simulink model "Vehicle_direction_detection"  (R2019a)
settings: Solver=FixedStepAuto  StartTime=0.0  StopTime=2000  FixedStep=0.01  RelTol=1e-3
libraries: simulink x6
settings Model: DataDictionary=Vehicle_Direction_Detection.sldd  Creator=賽維涅什  LastModifiedBy=賽維涅什
settings OptimizationCC: DefaultParameterBehavior=Inlined  EnhancedBackFolding=on  PassReuseOutputArgsAs=Individual arguments  OptimizeBlockOrder=speed  DifferentSizesBufferReuse=on  OptimizationCustomize=off
settings DebuggingCC: ParameterTunabilityLossMsg=error
settings SFSimCC: MATLABDynamicMemAlloc=off
settings RTWCC: SystemTargetFile=ert.tlc  GenCodeOnly=on  TemplateMakefile=ert_default_tmf  GenerateReport=on  IncludeHyperlinkInReport=on  LaunchReport=on  GenerateTraceInfo=on  GenerateTraceReport=on  GenerateTraceReportSl=on  GenerateTraceReportSf=on  GenerateTraceReportEml=on
settings CodeAppCC: ForceParamTrailComments=on  IgnoreCustomStorageClasses=off  OperatorAnnotations=on  SimulinkDataObjDesc=on  SFDataObjDesc=on  InsertBlockDesc=on
settings ERTTargetCC: TargetLangStandard=C99 (ISO)  GenerateSampleERTMain=on  InlinedParameterPlacement=NonHierarchical  ERTCustomFileTemplate=example_file_process.tlc

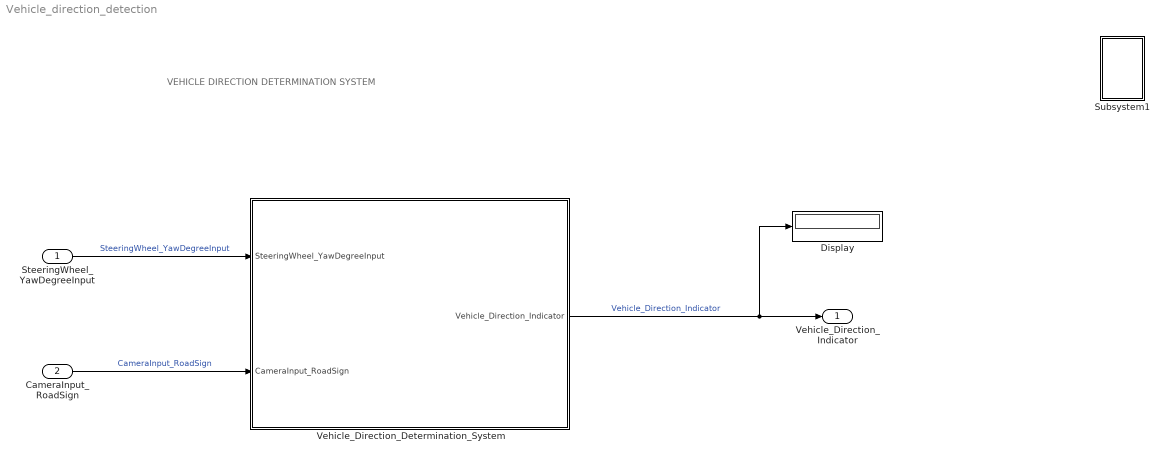
== system Vehicle_direction_detection ==
  note: VEHICLE DIRECTION DETERMINATION SYSTEM
  SteeringWheel_YawDegreeInput : Inport
  CameraInput_RoadSign : Inport  Port=2
  " Vehicle_Direction_Determination_System" : Subsystem
  Display : Display
  Subsystem1 : Subsystem
  Vehicle_Direction_Indicator : Outport
  wires:
  SteeringWheel_YawDegreeInput/1 -> " Vehicle_Direction_Determination_System"/1(SteeringWheel_YawDegreeInput)  "SteeringWheel_YawDegreeInput"
  CameraInput_RoadSign/1 -> " Vehicle_Direction_Determination_System"/2(CameraInput_RoadSign)  "CameraInput_RoadSign"
  " Vehicle_Direction_Determination_System"/1(Vehicle_Direction_Indicator) -> Display/1, Vehicle_Direction_Indicator/1  "Vehicle_Direction_Indicator"

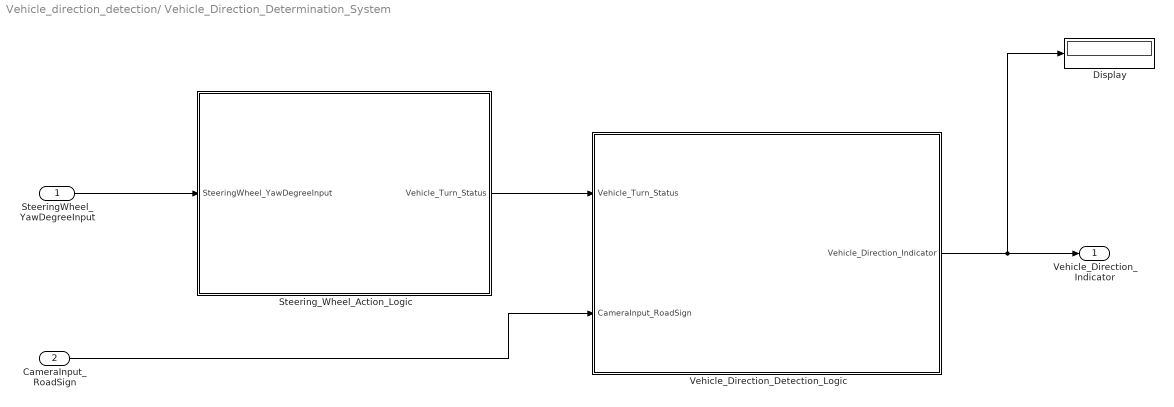
== system Vehicle_direction_detection/ Vehicle_Direction_Determination_System ==
  SteeringWheel_YawDegreeInput : Inport
  CameraInput_RoadSign : Inport  Port=2
  Display : Display
  Steering_Wheel_Action_Logic : Subsystem
  Vehicle_Direction_Detection_Logic : Subsystem
  Vehicle_Direction_Indicator : Outport
  wires:
  CameraInput_RoadSign/1 -> Vehicle_Direction_Detection_Logic/2(CameraInput_RoadSign)
  Vehicle_Direction_Detection_Logic/1(Vehicle_Direction_Indicator) -> Display/1, Vehicle_Direction_Indicator/1
  Steering_Wheel_Action_Logic/1(Vehicle_Turn_Status) -> Vehicle_Direction_Detection_Logic/1(Vehicle_Turn_Status)
  SteeringWheel_YawDegreeInput/1 -> Steering_Wheel_Action_Logic/1(SteeringWheel_YawDegreeInput)

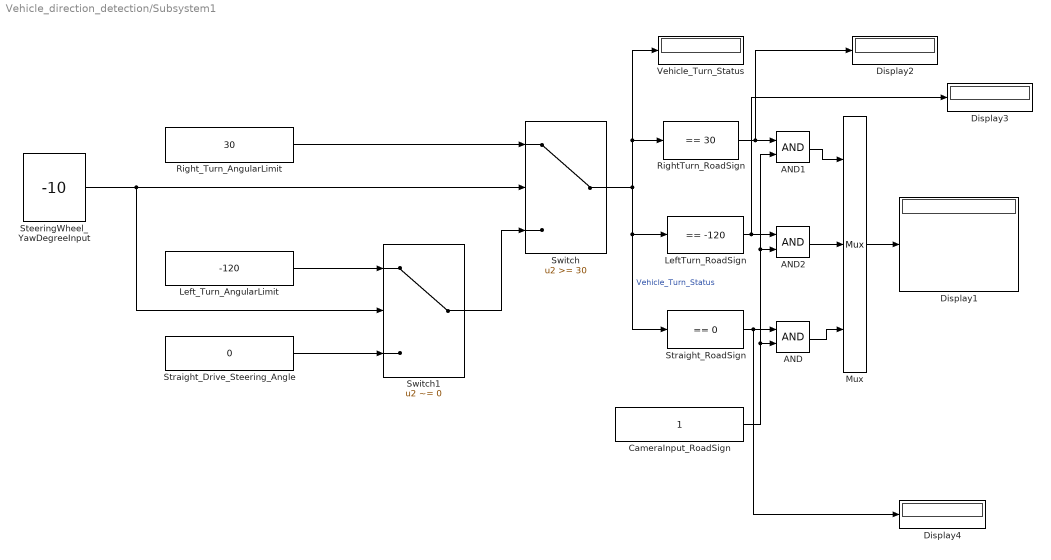
== system Vehicle_direction_detection/Subsystem1 ==
  AND : Logic  AllPortsSameDT=off  OutDataTypeStr=boolean
  AND1 : Logic  AllPortsSameDT=off  OutDataTypeStr=boolean
  AND2 : Logic  AllPortsSameDT=off  OutDataTypeStr=boolean
  CameraInput_RoadSign : Constant  OutMin=0  OutMax=1  OutDataTypeStr=boolean
  Display{1..4} (4 alike) : Display
  LeftTurn_RoadSign : simulink/Logic and Bit Operations/Compare To Constant  relop===  const=-120  OutDataTypeStr=boolean
  Left_Turn_AngularLimit : Constant  Value=-120  OutMin=-180  OutMax=180  OutDataTypeStr=int16
  Mux : Mux  Inputs=3
  RightTurn_RoadSign : simulink/Logic and Bit Operations/Compare To Constant  relop===  const=30  OutDataTypeStr=boolean
  Right_Turn_AngularLimit : Constant  Value=30  OutMin=-180  OutMax=180  OutDataTypeStr=int16
  SteeringWheel_YawDegreeInput : Constant  Value=-10  OutMin=-180  OutMax=180  OutDataTypeStr=int16
  Straight_Drive_Steering_Angle : Constant  Value=0  OutMin=-180  OutMax=180  OutDataTypeStr=int16
  Straight_RoadSign : simulink/Logic and Bit Operations/Compare To Constant  relop===  const=0  OutDataTypeStr=boolean
  Switch : Switch  Threshold=30
  Switch1 : Switch  Criteria=u2 ~= 0
  Vehicle_Turn_Status : Display
  wires:
  SteeringWheel_YawDegreeInput/1 -> Switch1/2, Switch/2
  Left_Turn_AngularLimit/1 -> Switch1/1
  Mux/1 -> Display1/1
  Switch/1 -> RightTurn_RoadSign/1, Vehicle_Turn_Status/1, Straight_RoadSign/1, LeftTurn_RoadSign/1  "Vehicle_Turn_Status"
  Straight_Drive_Steering_Angle/1 -> Switch1/3
  Right_Turn_AngularLimit/1 -> Switch/1
  Switch1/1 -> Switch/3
  AND1/1 -> Mux/1
  Straight_RoadSign/1 -> Display4/1, AND/1
  RightTurn_RoadSign/1 -> Display2/1, AND1/1
  CameraInput_RoadSign/1 -> AND1/2, AND2/2, AND/2
  AND/1 -> Mux/3
  LeftTurn_RoadSign/1 -> Display3/1, AND2/1
  AND2/1 -> Mux/2

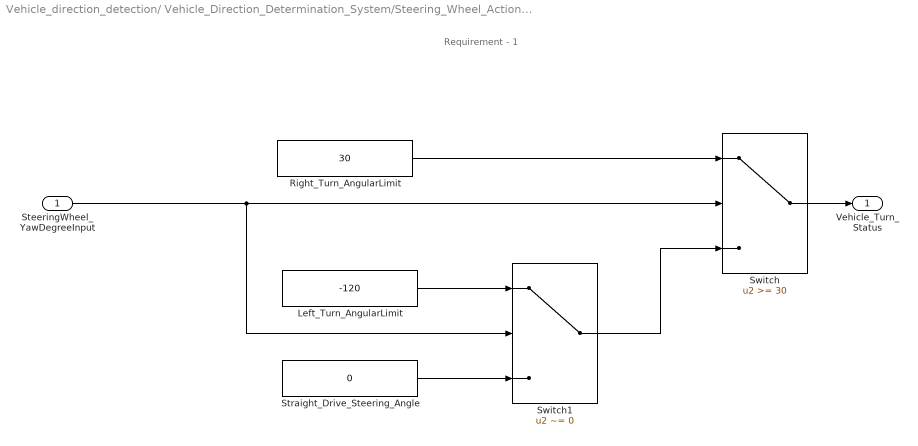
== system Vehicle_direction_detection/ Vehicle_Direction_Determination_System/Steering_Wheel_Action_Logic ==
  note: Requirement - 1
  SteeringWheel_YawDegreeInput : Inport
  Left_Turn_AngularLimit : Constant  Value=-120  OutMin=-180  OutMax=180  OutDataTypeStr=int16
  Right_Turn_AngularLimit : Constant  Value=30  OutMin=-180  OutMax=180  OutDataTypeStr=int16
  Straight_Drive_Steering_Angle : Constant  Value=0  OutMin=-180  OutMax=180  OutDataTypeStr=int16
  Switch : Switch  Threshold=30
  Switch1 : Switch  Criteria=u2 ~= 0
  Vehicle_Turn_Status : Outport
  wires:
  Right_Turn_AngularLimit/1 -> Switch/1
  Switch1/1 -> Switch/3
  Switch/1 -> Vehicle_Turn_Status/1
  Left_Turn_AngularLimit/1 -> Switch1/1
  SteeringWheel_YawDegreeInput/1 -> Switch1/2, Switch/2
  Straight_Drive_Steering_Angle/1 -> Switch1/3

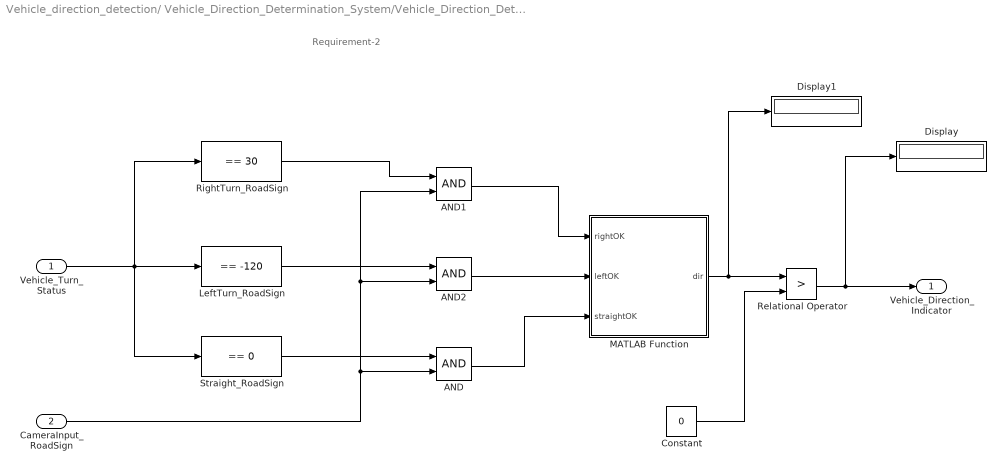
== system Vehicle_direction_detection/ Vehicle_Direction_Determination_System/Vehicle_Direction_Detection_Logic ==
  note: Requirement-2
  Vehicle_Turn_Status : Inport
  CameraInput_RoadSign : Inport  Port=2
  AND : Logic  AllPortsSameDT=off  OutDataTypeStr=boolean
  AND1 : Logic  AllPortsSameDT=off  OutDataTypeStr=boolean
  AND2 : Logic  AllPortsSameDT=off  OutDataTypeStr=boolean
  Constant : Constant  Value=0
  Display : Display
  Display1 : Display
  LeftTurn_RoadSign : simulink/Logic and Bit Operations/Compare To Constant  relop===  const=-120  OutDataTypeStr=boolean
  MATLAB Function : MATLAB Function  TreatAsAtomicUnit=on
  Relational Operator : RelationalOperator  Operator=>  OutDataTypeStr=boolean  RndMeth=Simplest
  RightTurn_RoadSign : simulink/Logic and Bit Operations/Compare To Constant  relop===  const=30  OutDataTypeStr=boolean
  Straight_RoadSign : simulink/Logic and Bit Operations/Compare To Constant  relop===  const=0  OutDataTypeStr=boolean
  Vehicle_Direction_Indicator : Outport
  wires:
  RightTurn_RoadSign/1 -> AND1/1
  CameraInput_RoadSign/1 -> AND/2, AND2/2, AND1/2
  Vehicle_Turn_Status/1 -> Straight_RoadSign/1, LeftTurn_RoadSign/1, RightTurn_RoadSign/1
  LeftTurn_RoadSign/1 -> AND2/1
  Straight_RoadSign/1 -> AND/1
  AND2/1 -> MATLAB Function/2(leftOK)
  AND1/1 -> MATLAB Function/1(rightOK)
  AND/1 -> MATLAB Function/3(straightOK)
  MATLAB Function/1(dir) -> Display1/1, Relational Operator/1
  Constant/1 -> Relational Operator/2
  Relational Operator/1 -> Display/1, Vehicle_Direction_Indicator/1

== matlab function Vehicle_direction_detection/ Vehicle_Direction_Determination_System/Vehicle_Direction_Detection_Logic/MATLAB Function ==
  data: rightOK input; leftOK input; straightOK input; dir output
function dir = getDirection(rightOK, leftOK, straightOK)
%#codegen
    dir = int8(0);  % Default: 0 = No direction
    if rightOK
        dir = int8(1);  % 1 = Right
    elseif leftOK
        dir = int8(2);  % 2 = Left
    elseif straightOK
        dir = int8(3);  % 3 = Straight
    end
end
